simulink model "robot_dynamics_model"  (R2019b)
settings: Solver=ode3  StartTime=0.0  StopTime=inf  FixedStep=0.005  RelTol=1e-3  EnableMultiTasking=on
values from neighbouring files (symbols this model uses):
  P = omega^2*tau/k    [PV_controller_TF.m]    (also in TransformPoints.m = P(1:3,:))
  V = (2*zeta*omega*tau-1)/k    [PV_controller_TF.m]
libraries: simulink x3
settings Model: ExtModeTrigDuration=5000  Creator=crbonney  LastModifiedBy=Chris
settings SolverCC: PositivePriorityOrder=on
settings DataIOCC: LimitDataPoints=on  SaveFormat=Array  ReturnWorkspaceOutputs=off
settings OptimizationCC: ExpressionDepthLimit=2147483647  LifeSpan=inf
settings DebuggingCC: UnderspecifiedInitializationDetection=Classic  MergeDetectMultiDrivingBlocksExec=none  SolverPrmCheckMsg=warning  StateNameClashWarn=warning  SFUnexpectedBacktrackingDiag=warning  SFNoUnconditionalDefaultTransitionDiag=warning  SFExecutionAtInitializationDiag=none  ArithmeticOperatorsInVariantConditions=warning
settings HardwareCC: ProdBitPerPointer=32  ProdBitPerSizeT=32  ProdBitPerPtrDiffT=32  ProdLargestAtomicFloat=None  ProdIntDivRoundTo=Undefined  ProdEndianess=Unspecified  ProdWordSize=32  ProdHWDeviceType=32-bit Generic
settings ModelReferenceCC: PropagateSignalLabelsOutOfModel=off
settings SFSimCC: SimUseLocalCustomCode=off  CustomCodeUndefinedFunction=UseInterfaceOnly
settings RTWCC: Description=QUARC Win64 Target  SystemTargetFile=quarc_win64.tlc  TemplateMakefile=quarc_default_tmf  RTWUseLocalCustomCode=off
settings CodeAppCC: StateflowObjectComments=on
settings STFCustomTargetCC: TargetPreCompLibLocation=C:\PROGRA~3\QUARC\lib\2012b\win64\release  GeneratePreprocessorConditionals=Disable all  CombineOutputUpdateFcns=on  CPPClassGenCompliant=on  SystemTargetFile=quarc_win64.tlc
settings GRTTargetCC: TargetPreCompLibLocation=C:\PROGRA~3\QUARC\lib\2012b\win64\release  TargetLangStandard=C89/C90 (ANSI)  ParMdlRefBuildCompliant=off  CompOptLevelCompliant=off  ConcurrentExecutionCompliant=off  GeneratePreprocessorConditionals=Disable all  MatFileLogging=off  UseToolchainInfoCompliant=off  ExtMode=on  ExtModeMexFile=quarc_comm
settings ConfigComp: CovMetricSettings=dw  CovHtmlReporting=on  CovSaveCumulativeToWorkspaceVar=on  CovSaveSingleToWorkspaceVar=on  CovExternalEMLEnable=off

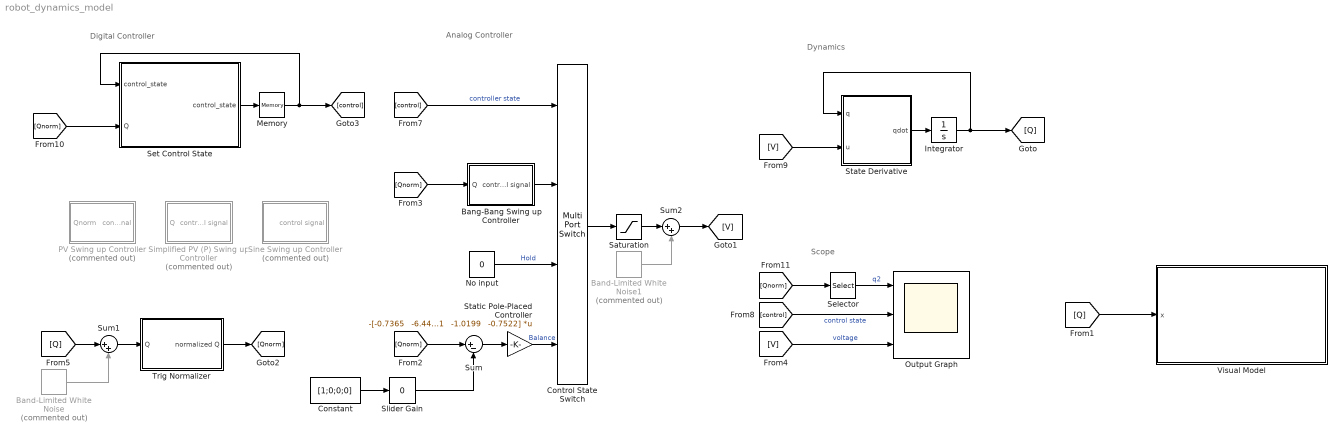
== system robot_dynamics_model ==
  note: Analog Controller
  note: Digital Controller
  note: Scope
  note: Dynamics
  " Static Pole-Placed Controller" : Gain  Gain="-[-0.7365   -6.4431   -1.0199   -0.7522]"  Multiplication=Matrix(K*u)
  Band-Limited White Noise : simulink/Sources/Band-Limited White Noise  Commented=on  Cov=0.00001*[1 1 100 100]  Ts=0.005  seed=[1 2 3 4]
  Band-Limited White Noise1 : simulink/Sources/Band-Limited White Noise  Commented=on  Cov=0.001  Ts=0.005  seed=[23341]
  Bang-Bang Swing up Controller : Subsystem
  Constant : Constant  Value=[1;0;0;0]
  Control State Switch : MultiPortSwitch
  Integrator : Integrator  InitialCondition=[0;pi;0;0.1]
  Memory : Memory  InitialCondition=3  InheritSampleTime=on
  No input : Constant  Value=0
  "Output Graph " : Scope  NumInputPorts=3
  PV Swing up Controller : Subsystem  Commented=on
  Saturation : Saturate  UpperLimit=10  LowerLimit=-10
  Selector : Selector  InputPortWidth=4  IndexOptions=Index vector (dialog)  Indices=[1 2]  OutputSizes=1
  Set Control State : MATLAB Function  TreatAsAtomicUnit=on
  Simplified PV (P) Swing up Controller : Subsystem  Commented=on
  Sine Swing up Controller : Subsystem  Commented=on
  Slider Gain : simulink/Math Operations/Slider Gain  gain=0  low=-3.14  high=3.14
  State Derivative : MATLAB Function  TreatAsAtomicUnit=on
  Sum : Sum  Inputs=|+-
  Sum1 : Sum  Inputs=|++
  Sum2 : Sum  Inputs=|++
  Trig Normalizer : Subsystem
  Visual Model : MATLAB Function  TreatAsAtomicUnit=on
  wires:
  Saturation/1 -> Sum2/1
  [Q] -> Visual Model/1(x)
  Integrator/1 -> [Q], State Derivative/1(q)
  No input/1 -> Control State Switch/3  "Hold"
  Set Control State/1(control_state) -> Memory/1
  [Qnorm] -> Set Control State/2(Q)
  Control State Switch/1 -> Saturation/1
  [V] -> "Output Graph "/3  "voltage"
  " Static Pole-Placed Controller"/1 -> Control State Switch/4  "Balance"
  [Qnorm] -> Sum/1
  [Q] -> Sum1/1
  Trig Normalizer/1(normalized Q) -> [Qnorm]
  Memory/1 -> Set Control State/1("control_state "), [control]
  [control] -> Control State Switch/1  "controller state"
  [control] -> "Output Graph "/2  "control state"
  Sum1/1 -> Trig Normalizer/1(Q)
  Band-Limited White Noise/1 -> Sum1/2
  Band-Limited White Noise1/1 -> Sum2/2
  Sum2/1 -> [V]
  [Qnorm] -> Bang-Bang Swing up Controller/1(Q)
  Bang-Bang Swing up Controller/1(control signal) -> Control State Switch/2
  [Qnorm] -> Selector/1
  Selector/1 -> "Output Graph "/1  "q2"
  [V] -> State Derivative/2(u)
  State Derivative/1(qdot) -> Integrator/1
  Constant/1 -> Slider Gain/1
  Sum/1 -> " Static Pole-Placed Controller"/1
  Slider Gain/1 -> Sum/2

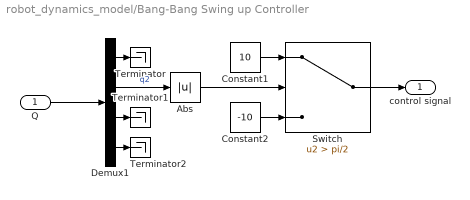
== system robot_dynamics_model/Bang-Bang Swing up Controller ==
  Q : Inport
  Abs : Abs
  Constant1 : Constant  Value=10
  Constant2 : Constant  Value=-10
  Demux1 : Demux
  Switch : Switch  Criteria=u2 > Threshold  Threshold=pi/2
  Terminator : Terminator
  Terminator1 : Terminator
  Terminator2 : Terminator
  control signal : Outport
  wires:
  Abs/1 -> Switch/2
  Q/1 -> Demux1/1
  Constant1/1 -> Switch/1
  Constant2/1 -> Switch/3
  Switch/1 -> control signal/1
  Demux1/1 -> Terminator/1
  Demux1/3 -> Terminator1/1
  Demux1/4 -> Terminator2/1
  Demux1/2 -> Abs/1  "q2"

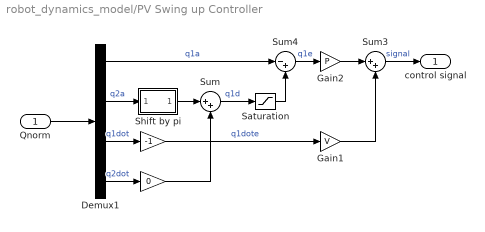
== system robot_dynamics_model/PV Swing up Controller ==
  Qnorm : Inport
  " " : Gain  Gain=-1
  "     " : Gain  Gain=0
  Demux1 : Demux
  Gain1 : Gain  Gain=V
  Gain2 : Gain  Gain=P
  Saturation : Saturate  UpperLimit=pi/6  LowerLimit=-pi/6
  Shift by pi : Subsystem
  Sum : Sum  Inputs=|++
  Sum3 : Sum  Inputs=|++
  Sum4 : Sum  Inputs=|-+
  control signal : Outport
  wires:
  Demux1/3 -> " "/1  "q1dot"
  Sum4/1 -> Gain2/1  "q1e"
  Qnorm/1 -> Demux1/1
  Gain1/1 -> Sum3/2
  Gain2/1 -> Sum3/1
  Sum3/1 -> control signal/1  "signal"
  Demux1/1 -> Sum4/1  "q1a"
  Demux1/4 -> "     "/1  "q2dot"
  Shift by pi/1(q2n) -> Sum/1
  Demux1/2 -> Shift by pi/1(q2)  "q2a"
  " "/1 -> Gain1/1  "q1dote"
  Sum/1 -> Saturation/1  "q1d"
  "     "/1 -> Sum/2
  Saturation/1 -> Sum4/2

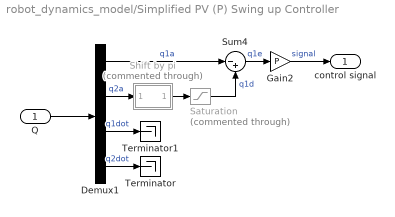
== system robot_dynamics_model/Simplified PV (P) Swing up Controller ==
  Q : Inport
  Demux1 : Demux
  Gain2 : Gain  Gain=P
  Saturation : Saturate  Commented=through  UpperLimit=pi/6  LowerLimit=-pi/6
  Shift by pi : Subsystem  Commented=through
  Sum4 : Sum  Inputs=|-+
  Terminator : Terminator
  Terminator1 : Terminator
  control signal : Outport
  wires:
  Shift by pi/1(q2n) -> Saturation/1
  Demux1/4 -> Terminator/1  "q2dot"
  Demux1/1 -> Sum4/1  "q1a"
  Gain2/1 -> control signal/1  "signal"
  Saturation/1 -> Sum4/2  "q1d"
  Demux1/2 -> Shift by pi/1(q2)  "q2a"
  Demux1/3 -> Terminator1/1  "q1dot"
  Q/1 -> Demux1/1
  Sum4/1 -> Gain2/1  "q1e"

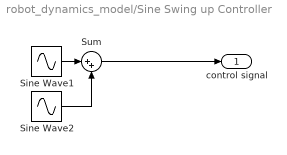
== system robot_dynamics_model/Sine Swing up Controller ==
  Sine Wave1 : Sin  Amplitude=5  Frequency=10
  Sine Wave2 : Sin  Amplitude=4.4  Frequency=15
  Sum : Sum  Inputs=|++
  control signal : Outport
  wires:
  Sine Wave2/1 -> Sum/2
  Sum/1 -> control signal/1
  Sine Wave1/1 -> Sum/1

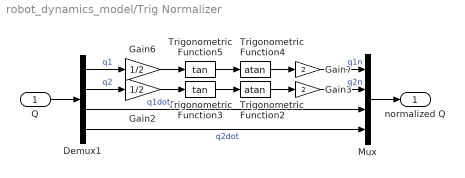
== system robot_dynamics_model/Trig Normalizer ==
  Q : Inport
  Demux1 : Demux
  Gain2 : Gain  Gain=1/2
  Gain3 : Gain  Gain=2
  Gain6 : Gain  Gain=1/2
  Gain7 : Gain  Gain=2
  Mux : Mux
  Trigonometric Function2 : Trigonometry  Operator=atan
  Trigonometric Function3 : Trigonometry  Operator=tan
  Trigonometric Function4 : Trigonometry  Operator=atan
  Trigonometric Function5 : Trigonometry  Operator=tan
  normalized Q : Outport
  wires:
  Trigonometric Function3/1 -> Trigonometric Function2/1
  Demux1/2 -> Gain2/1  "q2"
  Demux1/3 -> Mux/3  "q1dot"
  Demux1/4 -> Mux/4  "q2dot"
  Gain3/1 -> Mux/2  "q2n"
  Gain2/1 -> Trigonometric Function3/1
  Trigonometric Function2/1 -> Gain3/1
  Gain7/1 -> Mux/1  "q1n"
  Trigonometric Function4/1 -> Gain7/1
  Demux1/1 -> Gain6/1  "q1"
  Gain6/1 -> Trigonometric Function5/1
  Trigonometric Function5/1 -> Trigonometric Function4/1
  Q/1 -> Demux1/1
  Mux/1 -> normalized Q/1

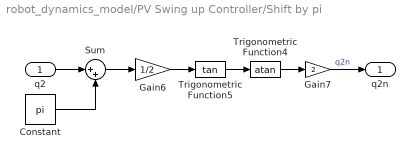
== system robot_dynamics_model/PV Swing up Controller/Shift by pi ==
  q2 : Inport
  Constant : Constant  Value=pi
  Gain6 : Gain  Gain=1/2
  Gain7 : Gain  Gain=2
  Sum : Sum  Inputs=|++
  Trigonometric Function4 : Trigonometry  Operator=atan
  Trigonometric Function5 : Trigonometry  Operator=tan
  q2n : Outport
  wires:
  Constant/1 -> Sum/2
  q2/1 -> Sum/1
  Trigonometric Function4/1 -> Gain7/1
  Gain6/1 -> Trigonometric Function5/1
  Trigonometric Function5/1 -> Trigonometric Function4/1
  Sum/1 -> Gain6/1
  Gain7/1 -> q2n/1  "q2n"

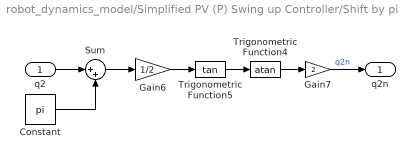
== system robot_dynamics_model/Simplified PV (P) Swing up Controller/Shift by pi ==
  q2 : Inport
  Constant : Constant  Value=pi
  Gain6 : Gain  Gain=1/2
  Gain7 : Gain  Gain=2
  Sum : Sum  Inputs=|++
  Trigonometric Function4 : Trigonometry  Operator=atan
  Trigonometric Function5 : Trigonometry  Operator=tan
  q2n : Outport
  wires:
  Constant/1 -> Sum/2
  q2/1 -> Sum/1
  Trigonometric Function4/1 -> Gain7/1
  Gain6/1 -> Trigonometric Function5/1
  Trigonometric Function5/1 -> Trigonometric Function4/1
  Sum/1 -> Gain6/1
  Gain7/1 -> q2n/1  "q2n"

== matlab function robot_dynamics_model/Visual Model ==
  data: x input
function ModelRobot (x)

theta1 = x(1);
theta2 = x(2);

frame0_links  = [...
        -.5 -.5 -.5 -.5 -.5  .5  .5 -.5  .5  .5 -.5  .5  .5 -.5  .5  .5;...
         .5 -.5 -.5  .5  .5  .5  .5  .5  .5 -.5 -.5 -.5 -.5 -.5 -.5  .5;...
        -15 -15 -.5 -.5 -15 -15 -.5 -.5 -.5 -.5 -.5 -.5 -15 -15 -15 -15;...
];

frame1_links = [...
         .5 -.5 -.5  .5  .5  .5  .5  .5  .5 -.5 -.5 -.5 -.5 -.5 -.5  .5;...
          8   8 -.5 -.5   8   8 -.5 -.5 -.5 -.5 -.5 -.5   8   8   8   8;...
        -.5 -.5 -.5 -.5 -.5  .5  .5 -.5  .5  .5 -.5  .5  .5 -.5  .5  .5;...
];
     
frame2_links = [...
         .2 -.2 -.2  .2  .2  .2  .2  .2  .2 -.2 -.2 -.2 -.2 -.2 -.2  .2;...
         12  12 -.5 -.5  12  12 -.5 -.5 -.5 -.5 -.5 -.5  12  12  12  12;...
        -.4 -.4 -.4 -.4 -.4   0   0 -.4   0   0 -.4   0   0 -.4   0   0;...
];

    rho = sqrt(8^2+12^2);
    phi_max = atan(12/8);

    f1 = TransformPoints(TRANS0_1(theta1),frame1_links);
    f2 = TransformPoints(TRANS0_1(theta1),TransformPoints(TRANS1_2(theta2),frame2_links));


    plot3(frame0_links(1,:),frame0_links(2,:), frame0_links(3,:),'bs-','LineWidth',3);
    axis([-15 15 -15 15 -15 15]);
    grid on
    hold on
    xlabel('x');
    ylabel('y');
    zlabel('z');
    plot3(f1(1,:),f1(2,:), f1(3,:),'rs-','LineWidth',3);
    plot3(f2(1,:),f2(2,:), f2(3,:),'go-', 'MarkerFaceColor', 'c', 'MarkerSize',5,'LineWidth',3);
    plot3(f2(1,end),f2(2,end), f2(3,end),'go-', 'MarkerFaceColor', 'c', 'MarkerSize',5,'LineWidth',3);
    axis([-15 15 -15 15 -15 15]);
%     WorkEnvelope2(rho, phi_max);
    hold off
end

== matlab function robot_dynamics_model/Set Control State ==
  data: control_state input; control_state output; Q input
function control_state = SetControlState(control_state, Q)

% q1 = Q(1);
q2 = Q(2);
q1dot = Q(3);
q2dot = Q(4);

q2 = 2*atan2(tan(q2/2),1);

switch control_state
    
    case 1
        if (abs(q2) <= 15*pi/180)
            control_state = 3;
        end
    case 2
        if (abs(q2) > pi-5*pi/180 && abs(q2dot) < 0.1 && abs(q1dot) < 0.1)
            control_state = 1;
        end
    case 3
        if abs(q2) > 25*pi/180
            control_state = 2;
        end
end

== matlab function robot_dynamics_model/State Derivative ==
  data: q input; u input; qdot output
function qdot = fcn(q, u)

%% constants
% J1 = 0.0012;
% m2 = 0.127;
% L12 = 0.2;
% L2 = 0.3;
% Lc2 = L2/2;
% beta1 = 0.015;
% beta2 = 0.002;
% Ra = 2.6;
% kt = 0.00768;
% kr = 70;
g = 9.81;
% 
%% parameters
% theta1 = (J1+m2*L12^2)*Ra/(kr*kt);
% theta2 = 1/3*m2*L2^2*Ra/(kr*kt);
% theta3 = 1/2*m2*L12*L2*Ra/(kr*kt);
% theta4 = m2*Lc2*Ra/(kr*kt);
% theta5 = beta1*Ra/(kr*kt)+kr*kt;
% theta6 = beta2*Ra/(kr*kt);
theta1 = 0.030372023809524;
theta2 = 0.018426339285714;
theta3 = 0.018426339285714;
theta4 = 0.092131696428571;
theta5 = 0.610144642857143;
theta6 = 0.009672619047619;

%% unpack vector
% q1 = q(1);
q2 = q(2);
q1dot = q(3);
q2dot = q(4);
v = [u; 0];

%% make matrices
m =    [...
        (theta1+theta2*sin(q2)^2)   (theta3*cos(q2)) ;...
            (theta3*cos(q2))            (theta2)     ;...
];


c =    [...
        (2*theta2*sin(q2)*cos(q2)*q2dot)     (-theta3*sin(q2)*q2dot) ;...
         (-theta2*sin(q2)*cos(q2)*q1dot)               (0)           ;...
];


f =    [...
         theta5*q1dot;...
         theta6*q2dot;...
];

g =    [...
                0         ;...
        -theta4*g*sin(q2) ;...
];

%% get accleration
acceleration = -m\(c*[q1dot;q2dot]+f+g-v);

%% get state derivative
qdot = [q1dot;q2dot;acceleration];
